simulink model "Testbed_ClosedLoopTracking"  (R2024b)
settings: Solver=VariableStepAuto  StartTime=0.0  StopTime=tf  RelTol=1e-3
values from neighbouring files (symbols this model uses):
  gamma1_initial = deg2rad(0)    [CMG_Testbed_Attitude_Control.m]
  gamma2_initial = deg2rad(0)    [CMG_Testbed_Attitude_Control.m]
  p1 = linspace(gamma1_min,gamma1_max,10)    [CMG_Testbed_Attitude_Control.m]
  p2 = linspace(gamma2_min,gamma2_max,10)    [CMG_Testbed_Attitude_Control.m]
undefined symbols (not defined in the file or in its folder): K1, K2, K3, K4
libraries: simulink_extras x5, cstblocks x1
settings Model: Creator=lanhi  LastModifiedBy=lanhi

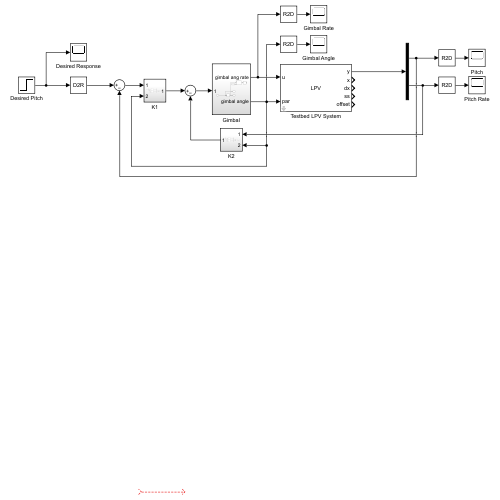
[thumbnail: Simulink's stored preview of the top-level diagram]
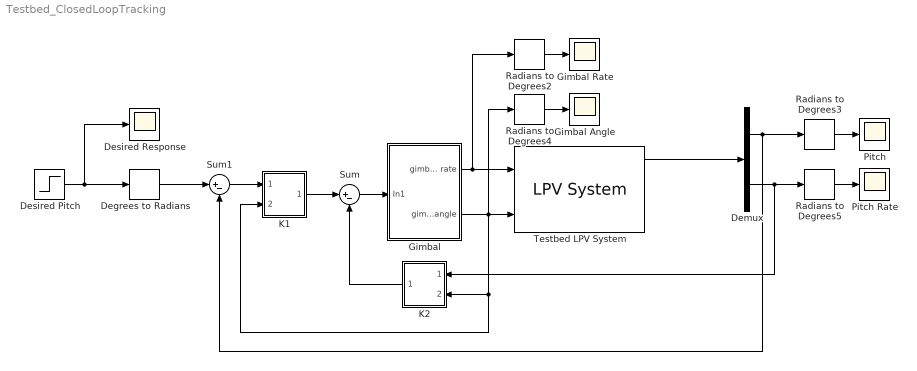
== system Testbed_ClosedLoopTracking ==
  Degrees to Radians : simulink_extras/Transformations/Degrees to Radians
  Demux : Demux  Outputs=2
  Desired Pitch : Step  After=20  SampleTime=0
  Desired Response : Scope
  Gimbal : Subsystem
  Gimbal Angle : Scope
  Gimbal Rate : Scope
  K1 : Subsystem
  K2 : Subsystem
  Pitch : Scope
  Pitch Rate : Scope
  Radians to Degrees{2..5} (4 alike) : simulink_extras/Transformations/Radians to Degrees
  Sum : Sum  Inputs=|+-
  Sum1 : Sum  Inputs=|+-
  Testbed LPV System : cstblocks/Linear Parameter Varying/LPV System  sys=ICs  InitialConditionSource=internal  InitialCondition=[deg2rad(0),0]  opSpecOption=Specify offsets as double arrays  uOffset=0  yOffset=0  xOffset=0  opEquilOption=on  dxOffset=0  AFixed=false  BFixed=false  CFixed=false  DFixed=false  uDelayFixed=false  yDelayFixed=false  iDelayFixed=false  sysFixedOption=First model in state-space array  sysFixed=[]  IMethod=Linear  EMethod=Clip  IndexSearch=Binary search  IndexBegin=on  OutputX=on  OutputXdot=on  OutputLTI=on  OutputOP=on  DataType=double  InitBufferSize=1024  FixedBuffer=off  SimMode=Interpreted execution  Offset=struct
  wires:
  ? -> ?
  Gimbal/2(gimbal angle) -> K1/2(In2), K2/2(In2), Testbed LPV System/2, Radians to Degrees4/1
  Testbed LPV System/1 -> Demux/1
  Radians to Degrees3/1 -> Pitch/1
  Desired Pitch/1 -> Desired Response/1, Degrees to Radians/1
  Degrees to Radians/1 -> Sum1/1
  Demux/1 -> Sum1/2, Radians to Degrees3/1
  Demux/2 -> K2/1(In1), Radians to Degrees5/1
  Radians to Degrees4/1 -> Gimbal Angle/1
  Sum1/1 -> K1/1(In1)
  K1/1(Out1) -> Sum/1
  K2/1(Out1) -> Sum/2
  Radians to Degrees2/1 -> Gimbal Rate/1
  Sum/1 -> Gimbal/1(In1)
  Gimbal/1(gimbal ang rate) -> Testbed LPV System/1, Radians to Degrees2/1
  Radians to Degrees5/1 -> Pitch Rate/1

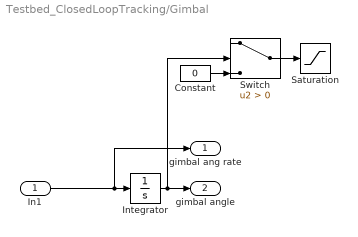
== system Testbed_ClosedLoopTracking/Gimbal ==
  In1 : Inport
  Constant : Constant  Value=0
  Integrator : Integrator  InitialCondition=[gamma1_initial,gamma2_initial]
  Saturation : Saturate
  Switch : Switch  Criteria=u2 > Threshold  SaturateOnIntegerOverflow=off  InputSameDT=off
  gimbal ang rate : Outport
  gimbal angle : Outport  Port=2
  wires:
  Integrator/1 -> gimbal angle/1, Switch/2
  In1/1 -> gimbal ang rate/1, Integrator/1
  Constant/1 -> Switch/3
  Switch/1 -> Saturation/1

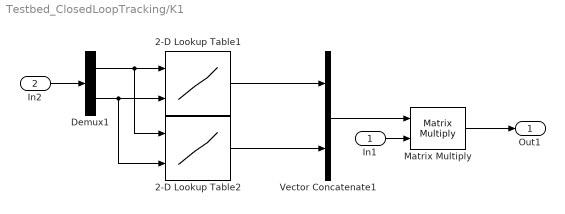
== system Testbed_ClosedLoopTracking/K1 ==
  In1 : Inport
  In2 : Inport  Port=2
  2-D Lookup Table1 : Lookup_n-D  BreakpointsForDimension1=p1  BreakpointsForDimension2=p2  Table=K1  InternalRulePriority=Speed  RndMeth=Simplest
      settings: InputPortMap=u0,u1
  2-D Lookup Table2 : Lookup_n-D  BreakpointsForDimension1=p1  BreakpointsForDimension2=p2  Table=K3  InternalRulePriority=Speed  RndMeth=Simplest
      settings: InputPortMap=u0,u1
  Demux1 : Demux  Outputs=2
  Matrix Multiply : Product  Multiplication=Matrix(*)
  Vector Concatenate1 : Concatenate
  Out1 : Outport
  wires:
  Demux1/1 -> 2-D Lookup Table2/1, 2-D Lookup Table1/1
  Vector Concatenate1/1 -> Matrix Multiply/1
  2-D Lookup Table2/1 -> Vector Concatenate1/2
  Demux1/2 -> 2-D Lookup Table2/2, 2-D Lookup Table1/2
  2-D Lookup Table1/1 -> Vector Concatenate1/1
  In2/1 -> Demux1/1
  In1/1 -> Matrix Multiply/2
  Matrix Multiply/1 -> Out1/1

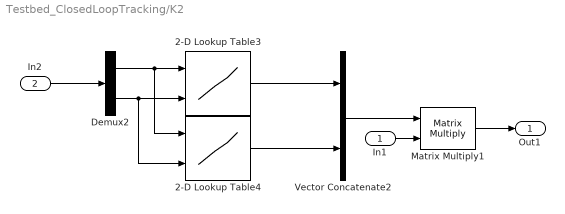
== system Testbed_ClosedLoopTracking/K2 ==
  In1 : Inport
  In2 : Inport  Port=2
  2-D Lookup Table3 : Lookup_n-D  BreakpointsForDimension1=p1  BreakpointsForDimension2=p2  Table=K2  InternalRulePriority=Speed  RndMeth=Simplest
      settings: InputPortMap=u0,u1
  2-D Lookup Table4 : Lookup_n-D  BreakpointsForDimension1=p1  BreakpointsForDimension2=p2  Table=K4  InternalRulePriority=Speed  RndMeth=Simplest
      settings: InputPortMap=u0,u1
  Demux2 : Demux  Outputs=2
  Matrix Multiply1 : Product  Multiplication=Matrix(*)
  Vector Concatenate2 : Concatenate
  Out1 : Outport
  wires:
  Demux2/1 -> 2-D Lookup Table4/1, 2-D Lookup Table3/1
  Demux2/2 -> 2-D Lookup Table4/2, 2-D Lookup Table3/2
  2-D Lookup Table4/1 -> Vector Concatenate2/2
  2-D Lookup Table3/1 -> Vector Concatenate2/1
  Vector Concatenate2/1 -> Matrix Multiply1/1
  Matrix Multiply1/1 -> Out1/1
  In2/1 -> Demux2/1
  In1/1 -> Matrix Multiply1/2
